simulink model "level27inverter"  (R2016a)
settings: Solver=ode23tb  StartTime=0.0  StopTime=4/50  MaxStep=1e-6  MinStep=1e-7  RelTol=1e-3
libraries: simulink x26, powerlib x18
settings Model: Creator=harikisan  LastModifiedBy=harikisan

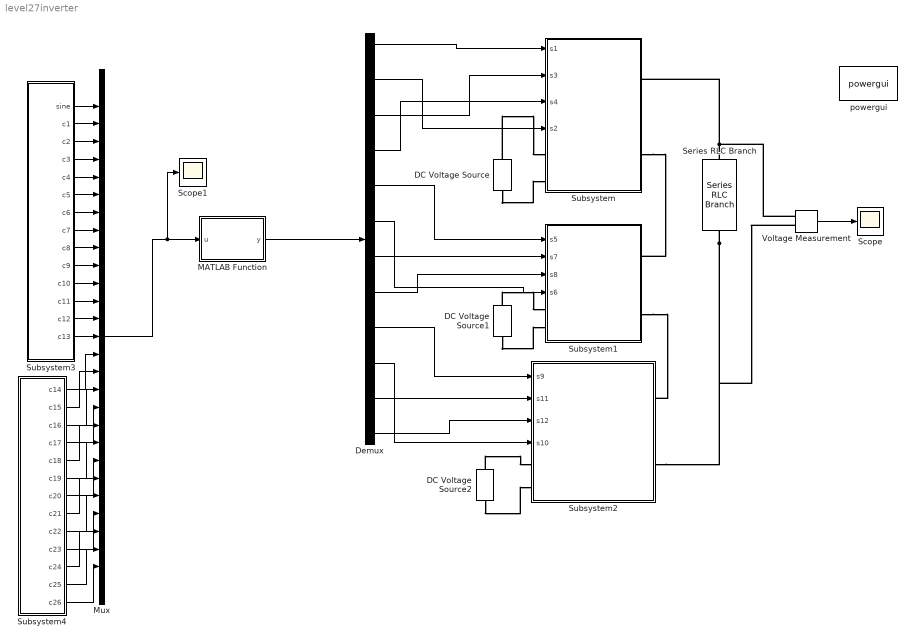
== system level27inverter ==
  DC Voltage Source : powerlib/Electrical Sources/DC Voltage Source  Amplitude=100  Measurements=None
  DC Voltage Source1 : powerlib/Electrical Sources/DC Voltage Source  Amplitude=300  Measurements=None
  DC Voltage Source2 : powerlib/Electrical Sources/DC Voltage Source  Amplitude=900  Measurements=None
  Demux : Demux  Outputs=12
  MATLAB Function : MATLAB Function  TreatAsAtomicUnit=on
  Mux : Mux  Inputs=27
  Scope : Scope
  Scope1 : Scope
  Series RLC Branch : powerlib/Elements/Series RLC Branch  LConnTagsString=__new0  RConnTagsString=__new0  BranchType=R  Resistance=100  Inductance=1e-3  SetiL0=off  InitialCurrent=0  Capacitance=1e-6  Setx0=off  InitialVoltage=0  Measurements=None
  Subsystem : Subsystem
  Subsystem1 : Subsystem
  Subsystem2 : Subsystem
  Subsystem3 : Subsystem
  Subsystem4 : Subsystem
  Voltage Measurement : powerlib/Measurements/Voltage Measurement  PhasorSimulation=off  OutputType=Complex  PSBequivalent=0
  powergui : powerlib/powergui  Priority=1  SimulationMode=Continuous  SolverType=Tustin/Backward Euler (TBE)  SampleTime=50e-6  frequency=60  SPID=off  DisableSnubberDevices=off  DisableRonSwitches=off  DisableVfSwitches=off  SwTol=0  DisplayEquations=off  Interpol=off  ExternalGateDelay=off  methode=off  Ts=10  FunctionMessages=off  echomessages=off  HookPort=off  EnableUseOfTLC=off  x0status=blocks  frequencyindice=0  Pbase=100e6  ErrMax=1e-4  Iterations=50  UnitsV=kV  UnitsW=MW  buscounter=0  RestoreLinks=warning  ResistiveCurrentMeasurement=off  Frange=[0:2:500]  Ylog=off  Xlog=on  ShowGrid=off  save=off  variable=ZData  structure=load27  ZoomFFT=off  StartTime=0.04  cycles=1  DisplayStyle=1  fundamental=50  FreqAxis=on  MaxFrequency=10000  frequencyindicesteady=1  RmsSteady=1  display=off
  wires:
  Voltage Measurement/1 -> Scope/1
  Demux/1 -> Subsystem/1(s1)
  Demux/2 -> Subsystem/4(s2)
  Demux/3 -> Subsystem/2(s3)
  Demux/4 -> Subsystem/3(s4)
  Demux/5 -> Subsystem1/1(s5)
  Demux/6 -> Subsystem1/4(s6)
  Demux/7 -> Subsystem1/2(s7)
  Demux/8 -> Subsystem1/3(s8)
  Demux/9 -> Subsystem2/1(s9)
  Demux/10 -> Subsystem2/4(s10)
  Demux/11 -> Subsystem2/2(s11)
  Demux/12 -> Subsystem2/3(s12)
  MATLAB Function/1(y) -> Demux/1
  Subsystem3/1(sine) -> Mux/1
  Subsystem3/2(c1) -> Mux/2
  Subsystem3/3(c2) -> Mux/3
  Subsystem3/4(c3) -> Mux/4
  Subsystem3/5(c4) -> Mux/5
  Subsystem3/6(c5) -> Mux/6
  Subsystem3/7(c6) -> Mux/7
  Subsystem3/8(c7) -> Mux/8
  Subsystem3/9(c8) -> Mux/9
  Subsystem3/10(c9) -> Mux/10
  Subsystem3/11(c10) -> Mux/11
  Subsystem3/12(c11) -> Mux/12
  Subsystem3/13(c12) -> Mux/13
  Subsystem3/14(c13) -> Mux/14
  Subsystem4/1(c14) -> Mux/15
  Subsystem4/2(c15) -> Mux/16
  Subsystem4/3(c16) -> Mux/17
  Subsystem4/4(c17) -> Mux/18
  Subsystem4/5(c18) -> Mux/19
  Subsystem4/6(c19) -> Mux/20
  Subsystem4/7(c20) -> Mux/21
  Subsystem4/8(c21) -> Mux/22
  Subsystem4/9(c22) -> Mux/23
  Subsystem4/10(c23) -> Mux/24
  Subsystem4/11(c24) -> Mux/25
  Subsystem4/12(c25) -> Mux/26
  Subsystem4/13(c26) -> Mux/27
  Mux/1 -> Scope1/1, MATLAB Function/1(u)
  connections:
  Voltage Measurement/LConn1 -- Series RLC Branch/LConn1 -- Subsystem/RConn1
  Series RLC Branch/RConn1 -- Subsystem2/RConn2 -- Voltage Measurement/LConn2
  DC Voltage Source1/RConn1 -- Subsystem1/LConn1
  DC Voltage Source2/RConn1 -- Subsystem2/LConn1
  DC Voltage Source1/LConn1 -- Subsystem1/LConn2
  DC Voltage Source/LConn1 -- Subsystem/LConn2
  DC Voltage Source2/LConn1 -- Subsystem2/LConn2
  Subsystem/RConn2 -- Subsystem1/RConn1
  DC Voltage Source/RConn1 -- Subsystem/LConn1
  Subsystem1/RConn2 -- Subsystem2/RConn1

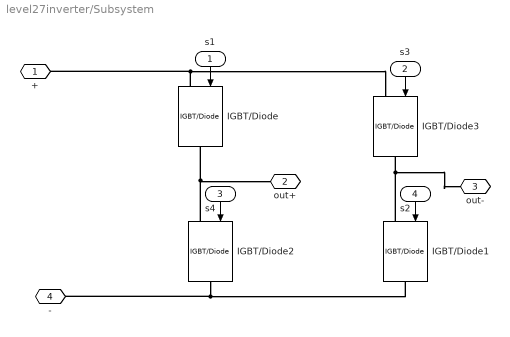
== system level27inverter/Subsystem ==
  s1 : Inport
  s3 : Inport  Port=2
  s4 : Inport  Port=3
  s2 : Inport  Port=4
  IGBT/Diode{,1..3} (4 alike) : powerlib/Power Electronics/IGBT//Diode  Ron=1e-3  Rs=1e5  Cs=inf  Measurements=off
  + : PMIOPort  Port=1  Side=Left
  out+ : PMIOPort  Port=2  Side=Right
  out- : PMIOPort  Port=3  Side=Right
  "- " : PMIOPort  Port=4  Side=Left
  wires:
  s4/1 -> IGBT/Diode2/1
  s1/1 -> IGBT/Diode/1
  s2/1 -> IGBT/Diode1/1
  s3/1 -> IGBT/Diode3/1
  connections:
  IGBT/Diode/LConn1 -- +/RConn1 -- IGBT/Diode3/LConn1
  IGBT/Diode2/LConn1 -- out+/RConn1 -- IGBT/Diode/RConn1
  IGBT/Diode1/LConn1 -- out-/RConn1 -- IGBT/Diode3/RConn1
  IGBT/Diode2/RConn1 -- "- "/RConn1 -- IGBT/Diode1/RConn1

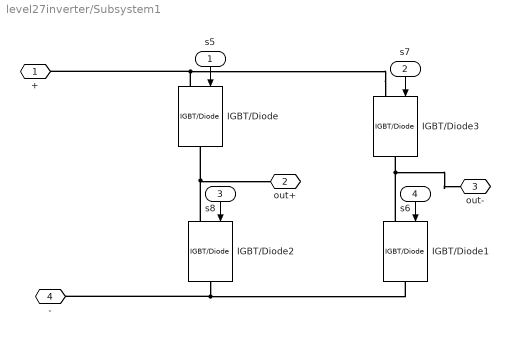
== system level27inverter/Subsystem1 ==
  s5 : Inport
  s7 : Inport  Port=2
  s8 : Inport  Port=3
  s6 : Inport  Port=4
  IGBT/Diode{,1..3} (4 alike) : powerlib/Power Electronics/IGBT//Diode  Ron=1e-3  Rs=1e5  Cs=inf  Measurements=off
  + : PMIOPort  Port=1  Side=Left
  out+ : PMIOPort  Port=2  Side=Right
  out- : PMIOPort  Port=3  Side=Right
  "- " : PMIOPort  Port=4  Side=Left
  wires:
  s8/1 -> IGBT/Diode2/1
  s5/1 -> IGBT/Diode/1
  s6/1 -> IGBT/Diode1/1
  s7/1 -> IGBT/Diode3/1
  connections:
  IGBT/Diode3/LConn1 -- IGBT/Diode/LConn1 -- +/RConn1
  IGBT/Diode/RConn1 -- IGBT/Diode2/LConn1 -- out+/RConn1
  IGBT/Diode1/LConn1 -- IGBT/Diode3/RConn1 -- out-/RConn1
  IGBT/Diode1/RConn1 -- IGBT/Diode2/RConn1 -- "- "/RConn1

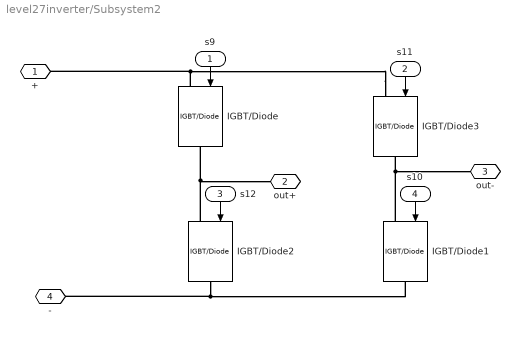
== system level27inverter/Subsystem2 ==
  s9 : Inport
  s11 : Inport  Port=2
  s12 : Inport  Port=3
  s10 : Inport  Port=4
  IGBT/Diode{,1..3} (4 alike) : powerlib/Power Electronics/IGBT//Diode  Ron=1e-3  Rs=1e5  Cs=inf  Measurements=off
  + : PMIOPort  Port=1  Side=Left
  out+ : PMIOPort  Port=2  Side=Right
  out- : PMIOPort  Port=3  Side=Right
  "- " : PMIOPort  Port=4  Side=Left
  wires:
  s12/1 -> IGBT/Diode2/1
  s9/1 -> IGBT/Diode/1
  s10/1 -> IGBT/Diode1/1
  s11/1 -> IGBT/Diode3/1
  connections:
  IGBT/Diode3/LConn1 -- IGBT/Diode/LConn1 -- +/RConn1
  IGBT/Diode/RConn1 -- IGBT/Diode2/LConn1 -- out+/RConn1
  IGBT/Diode1/LConn1 -- IGBT/Diode3/RConn1 -- out-/RConn1
  IGBT/Diode1/RConn1 -- IGBT/Diode2/RConn1 -- "- "/RConn1

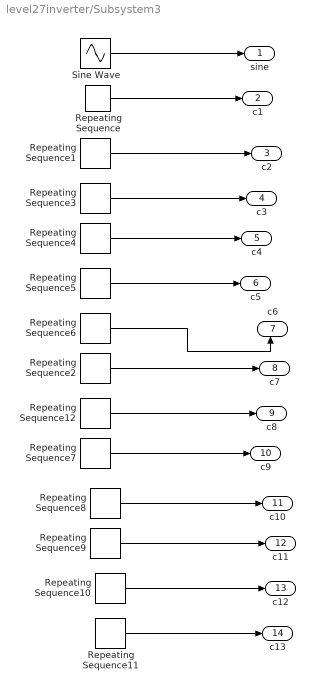
== system level27inverter/Subsystem3 ==
  Repeating Sequence : simulink/Sources/Repeating Sequence  rep_seq_t=[0 1/10000 1/5000]  rep_seq_y=[0 1 0]
  Repeating Sequence1 : simulink/Sources/Repeating Sequence  rep_seq_t=[0 1/10000 1/5000]  rep_seq_y=[1 2 1]
  Repeating Sequence10 : simulink/Sources/Repeating Sequence  rep_seq_t=[0 1/10000 1/5000]  rep_seq_y=[11 12 11]
  Repeating Sequence11 : simulink/Sources/Repeating Sequence  rep_seq_t=[0 1/10000 1/5000]  rep_seq_y=[12 13 12]
  Repeating Sequence12 : simulink/Sources/Repeating Sequence  rep_seq_t=[0 1/10000 1/5000]  rep_seq_y=[7 8 7]
  Repeating Sequence2 : simulink/Sources/Repeating Sequence  rep_seq_t=[0 1/10000 1/5000]  rep_seq_y=[6 7 6]
  Repeating Sequence3 : simulink/Sources/Repeating Sequence  rep_seq_t=[0 1/10000 1/5000]  rep_seq_y=[2 3 2]
  Repeating Sequence4 : simulink/Sources/Repeating Sequence  rep_seq_t=[0 1/10000 1/5000]  rep_seq_y=[3 4 3]
  Repeating Sequence5 : simulink/Sources/Repeating Sequence  rep_seq_t=[0 1/10000 1/5000]  rep_seq_y=[4 5 4]
  Repeating Sequence6 : simulink/Sources/Repeating Sequence  rep_seq_t=[0 1/10000 1/5000]  rep_seq_y=[5 6 5]
  Repeating Sequence7 : simulink/Sources/Repeating Sequence  rep_seq_t=[0 1/10000 1/5000]  rep_seq_y=[8 9 8]
  Repeating Sequence8 : simulink/Sources/Repeating Sequence  rep_seq_t=[0 1/10000 1/5000]  rep_seq_y=[9 10 9]
  Repeating Sequence9 : simulink/Sources/Repeating Sequence  rep_seq_t=[0 1/10000 1/5000]  rep_seq_y=[10 11 10]
  Sine Wave : Sin  Amplitude=13  Frequency=2*pi*50  SampleTime=0
  sine : Outport
  c1 : Outport  Port=2
  c2 : Outport  Port=3
  c3 : Outport  Port=4
  c4 : Outport  Port=5
  c5 : Outport  Port=6
  c6 : Outport  Port=7
  c7 : Outport  Port=8
  c8 : Outport  Port=9
  c9 : Outport  Port=10
  c10 : Outport  Port=11
  c11 : Outport  Port=12
  c12 : Outport  Port=13
  c13 : Outport  Port=14
  wires:
  Repeating Sequence/1 -> c1/1
  Repeating Sequence6/1 -> c6/1
  Repeating Sequence5/1 -> c5/1
  Repeating Sequence12/1 -> c8/1
  Repeating Sequence8/1 -> c10/1
  Repeating Sequence4/1 -> c4/1
  Repeating Sequence11/1 -> c13/1
  Repeating Sequence9/1 -> c11/1
  Repeating Sequence10/1 -> c12/1
  Sine Wave/1 -> sine/1
  Repeating Sequence7/1 -> c9/1
  Repeating Sequence1/1 -> c2/1
  Repeating Sequence3/1 -> c3/1
  Repeating Sequence2/1 -> c7/1

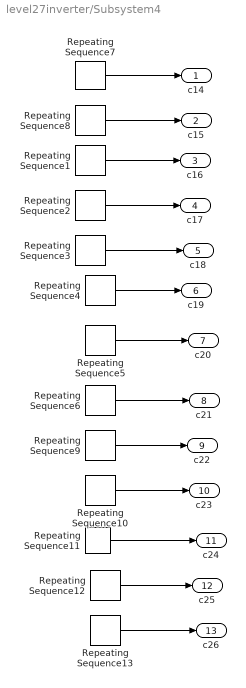
== system level27inverter/Subsystem4 ==
  Repeating Sequence1 : simulink/Sources/Repeating Sequence  rep_seq_t=[0 1/10000 1/5000]  rep_seq_y=[-2 -3 -2]
  Repeating Sequence10 : simulink/Sources/Repeating Sequence  rep_seq_t=[0 1/10000 1/5000]  rep_seq_y=[-9 -10 -9]
  Repeating Sequence11 : simulink/Sources/Repeating Sequence  rep_seq_t=[0 1/10000 1/5000]  rep_seq_y=[-10 -11 -10]
  Repeating Sequence12 : simulink/Sources/Repeating Sequence  rep_seq_t=[0 1/10000 1/5000]  rep_seq_y=[-11 -12 -11]
  Repeating Sequence13 : simulink/Sources/Repeating Sequence  rep_seq_t=[0 1/10000 1/5000]  rep_seq_y=[-12 -13 -12]
  Repeating Sequence2 : simulink/Sources/Repeating Sequence  rep_seq_t=[0 1/10000 1/5000]  rep_seq_y=[-3 -4 -3]
  Repeating Sequence3 : simulink/Sources/Repeating Sequence  rep_seq_t=[0 1/10000 1/5000]  rep_seq_y=[-4 -5 -4]
  Repeating Sequence4 : simulink/Sources/Repeating Sequence  rep_seq_t=[0 1/10000 1/5000]  rep_seq_y=[-5 -6 -5]
  Repeating Sequence5 : simulink/Sources/Repeating Sequence  rep_seq_t=[0 1/10000 1/5000]  rep_seq_y=[-6 -7 -6]
  Repeating Sequence6 : simulink/Sources/Repeating Sequence  rep_seq_t=[0 1/10000 1/5000]  rep_seq_y=[-7 -8 -7]
  Repeating Sequence7 : simulink/Sources/Repeating Sequence  rep_seq_t=[0 1/10000 1/5000]  rep_seq_y=[0 -1 0]
  Repeating Sequence8 : simulink/Sources/Repeating Sequence  rep_seq_t=[0 1/10000 1/5000]  rep_seq_y=[-1 -2 -1]
  Repeating Sequence9 : simulink/Sources/Repeating Sequence  rep_seq_t=[0 1/10000 1/5000]  rep_seq_y=[-8 -9 -8]
  c14 : Outport
  c15 : Outport  Port=2
  c16 : Outport  Port=3
  c17 : Outport  Port=4
  c18 : Outport  Port=5
  c19 : Outport  Port=6
  c20 : Outport  Port=7
  c21 : Outport  Port=8
  c22 : Outport  Port=9
  c23 : Outport  Port=10
  c24 : Outport  Port=11
  c25 : Outport  Port=12
  c26 : Outport  Port=13
  wires:
  Repeating Sequence10/1 -> c23/1
  Repeating Sequence1/1 -> c16/1
  Repeating Sequence8/1 -> c15/1
  Repeating Sequence4/1 -> c19/1
  Repeating Sequence6/1 -> c21/1
  Repeating Sequence9/1 -> c22/1
  Repeating Sequence13/1 -> c26/1
  Repeating Sequence11/1 -> c24/1
  Repeating Sequence3/1 -> c18/1
  Repeating Sequence2/1 -> c17/1
  Repeating Sequence12/1 -> c25/1
  Repeating Sequence5/1 -> c20/1
  Repeating Sequence7/1 -> c14/1

== matlab function level27inverter/MATLAB Function ==
  data: u input; y output
function y = fcn(u)

sine = u(1);

c1 = u(2);
c2 = u(3);
c3 = u(4);
c4 = u(5);
c5 = u(6);
c6 = u(7);
c7 = u(8);
c8 = u(9);
c9 = u(10);
c10 = u(11);
c11= u(12);
c12= u(13);
c13 = u(14);

c14 = u(15);
c15 = u(16);
c16 = u(17);
c17 = u(18);
c18 = u(19);
c19 = u(20);
c20 = u(21);
c21 = u(22);
c22 = u(23);
c23 = u(24);
c24 = u(25);
c25 = u(26);
c26 = u(27);

s1 = 0;
s3 = 0;
s5 = 0;
s7 = 0;
s2 = 0;
s4 = 0;
s6 = 0;
s8 = 0;
s9 = 0;
s10 = 0;
s11 = 0;
s12 = 0;

if (sine >= 0 && sine < 1)
    if (sine >= c1)
        s1 = 1;s2=1;s5=1;s7=1;s9=1;s11=1;
    else
        s1 = 1;s3=1;s5=1;s7=1;s9=1;s11=1;
    end
end

if (sine >= 1 && sine < 2)
    if (sine >= c2)
        s3 = 1;s4=1;s5=1;s6=1;s9=1;s11=1;
    else
         s1 = 1;s2=1;s5=1;s7=1;s9=1;s11=1;
    end
end

if (sine >= 2 && sine < 3)
    if (sine >= c3)
        s1 = 1;s3=1;s5=1;s6=1;s9=1;s11=1;
    else
        s3 = 1;s4=1;s5=1;s6=1;s9=1;s11=1;
    end
end

if (sine >= 3 && sine < 4)
    if (sine >= c4)
        s1 = 1;s2=1;s5=1;s6=1;s9=1;s11=1;
    else
         s1 = 1;s3=1;s5=1;s6=1;s9=1;s11=1;
    end
end

if (sine >= 4 && sine < 5)
    if (sine >= c5)
        s3 = 1;s4=1;s8=1;s7=1;s10=1;s9=1;
    else
        s1 = 1;s2=1;s5=1;s6=1;s9=1;s11=1;
    end
end

if (sine >= 5 && sine < 6)
    if (sine >= c6)
        s1 = 1;s3=1;s7=1;s8=1;s9=1;s10=1;
    else
       s3 = 1;s4=1;s8=1;s7=1;s10=1;s9=1;
    end
end

if (sine >= 6 && sine < 7)
    if (sine >= c7)
        s1 = 1;s2=1;s7=1;s8=1;s9=1;s10=1;
    else
        s1 = 1;s3=1;s7=1;s8=1;s9=1;s10=1;
    end
end

if (sine >= 7 && sine < 8)
    if (sine >= c8)
        s3 = 1;s4=1;s5=1;s7=1;s9=1;s10=1;
    else
        s1 = 1;s2=1;s7=1;s8=1;s9=1;s10=1;
    end
end

if (sine >= 8 && sine < 9)
    if (sine >= c9)
        s1 = 1;s3=1;s5=1;s7=1;s9=1;s10=1;
    else
        s3 = 1;s4=1;s5=1;s7=1;s9=1;s10=1;
    end
end

if (sine >= 9 && sine < 10)
    if (sine >= c10)
        s1 = 1;s2=1;s5=1;s7=1;s9=1;s10=1;
    else
        s1 = 1;s3=1;s5=1;s7=1;s9=1;s10=1;
    end
end

if (sine >= 10 && sine < 11)
    if (sine >= c11)
        s3 = 1;s4=1;s5=1;s6=1;s9=1;s10=1;
    else
        s1 = 1;s2=1;s5=1;s7=1;s9=1;s10=1;
    end
end

if (sine >= 11 && sine < 12)
    if (sine >= c12)
        s1 = 1;s3=1;s5=1;s6=1;s9=1;s10=1;
    else
        s3 = 1;s4=1;s5=1;s6=1;s9=1;s10=1;
    end
end

if (sine >= 12 && sine <= 13)
    if (sine >= c13)
        s1 = 1;s2=1;s5=1;s6=1;s9=1;s10=1;
    else
        s1 = 1;s3=1;s5=1;s6=1;s9=1;s10=1;
    end
end

if (sine < 0 && sine >= -1)
    if (sine <= c14)
        s3 = 1;s4=1;s5=1;s7=1;s9=1;s11=1;
    else
        s1 = 1;s3=1;s5=1;s7=1;s9=1;s11=1;
    end
end

if (sine < -1 && sine >= -2)
    if (sine <= c15)
        s1= 1;s2=1;s8=1;s7=1;s9=1;s11=1;
    else
         s3 = 1;s4=1;s5=1;s7=1;s9=1;s11=1;
    end
end

if (sine < -2 && sine >= -3)
    if (sine <= c16)
        s1= 1;s3=1;s8=1;s7=1;s9=1;s11=1;
    else
          s1= 1;s2=1;s8=1;s7=1;s9=1;s11=1;
    end
end

if (sine < -3 && sine >= -4)
    if (sine <= c17)
        s4 = 1;s3=1;s8=1;s7=1;s9=1;s11=1;
    else
        s1= 1;s3=1;s8=1;s7=1;s9=1;s11=1;
    end
end

if (sine < -4 && sine >= -5)
    if (sine <= c18)
        s1 = 1;s2=1;s5=1;s6=1;s12=1;s11=1;
    else
        s4 = 1;s3=1;s8=1;s7=1;s9=1;s11=1;
    end
end

if (sine < -5 && sine > -6)
    if (sine <= c19)
        s1 = 1;s3=1;s5=1;s6=1;s12=1;s11=1;
    else
        s1 = 1;s2=1;s5=1;s6=1;s12=1;s11=1;
    end
end

if (sine < -6 && sine >= -7)
    if (sine <= c20)
        s4 = 1;s3=1;s5=1;s6=1;s12=1;s11=1;
    else
        s1 = 1;s3=1;s5=1;s6=1;s12=1;s11=1;
    end
end

if (sine < -7 && sine >= -8)
    if (sine <= c21)
        s1 = 1;s2=1;s5=1;s7=1;s12=1;s11=1;
    else
        s4 = 1;s3=1;s5=1;s6=1;s12=1;s11=1;
    end
end

if (sine < -8 && sine >= -9)
    if (sine <= c22)
        s1= 1;s3=1;s5=1;s7=1;s12=1;s11=1;
    else
        s1 = 1;s2=1;s5=1;s7=1;s12=1;s11=1;
    end
end

if (sine < -9  &&  sine >= -10)
    if (sine <= c23)
        s3= 1;s4=1;s5=1;s7=1;s12=1;s11=1;
    else
          s1= 1;s3=1;s5=1;s7=1;s12=1;s11=1;
    end
end

if (sine < -10 && sine >= -11)
    if (sine <= c24)
        s1 = 1;s2=1;s8=1;s7=1;s12=1;s11=1;
    else
        s3= 1;s4=1;s5=1;s7=1;s12=1;s11=1;
    end
end

if (sine < -11 && sine >= -12)
    if (sine <= c25)
        s1 = 1;s3=1;s8=1;s7=1;s12=1;s11=1;
    else
         s1 = 1;s2=1;s8=1;s7=1;s12=1;s11=1;
    end
end

if (sine < -12 && sine >= -13)
    if (sine <= c26)
        s4 = 1;s3=1;s7=1;s8=1;s12=1;s11=1;
    else
        s1 = 1;s3=1;s8=1;s7=1;s12=1;s11=1;
    end
end

y = [s1; s2; s3; s4; s5; s6; s7; s8; s9; s10; s11; s12];
